simulink model "bmw_vehicle_dynamics"  (R2022b)
settings: Solver=ode45  StartTime=0.0  StopTime=10  RelTol=1e-3  EnableMultiTasking=on
PreLoadFcn:
  | % Execute script to load parameters
  | bmwParams;
values from neighbouring files (symbols this model uses):
  CD = 0.3    [ballParams.m]    (also in bmwParams.m = 0.4; bungeeParams.m = 0.6)
  Fdrive = 1000    [bmwParams.m]
  h = 4.15    [bmwParams.m]
  m = 0.145    [ballParams.m]    (also in bmwParams.m = 104.2; bungeeParams.m = 90)
  rho = 1.2    [ballParams.m]    (also in bmwParams.m = 0.002377; bungeeParams.m)
  w = 5.71    [bmwParams.m]    (also in manifold_press_start.mat = [209.48 209.479999353 209.479996118 209.479979943 209.479899; manifold_pressure.mat = [209.48 209.479999353 209.479996118 209.479979943 209.479899)
settings Model: Creator=jrivitus  LastModifiedBy=bensweet
settings SolverCC: AlgebraicLoopSolver=TrustRegion
settings DataIOCC: LimitDataPoints=on  SaveFormat=Array  ReturnWorkspaceOutputs=off
settings OptimizationCC: ExpressionDepthLimit=2147483647  LifeSpan=inf
settings DebuggingCC: UnderspecifiedInitializationDetection=Classic  MergeDetectMultiDrivingBlocksExec=none  ParameterPrecisionLossMsg=none  FcnCallInpInsideContextMsg=warning  UnconnectedInputMsg=warning  UnconnectedOutputMsg=warning  UnconnectedLineMsg=warning  AllowSymbolicDim=off  StateNameClashWarn=warning  PregeneratedLibrarySubsystemCodeDiagnostic=none  SFUnexpectedBacktrackingDiag=warning  SFNoUnconditionalDefaultTransitionDiag=warning  SFExecutionAtInitializationDiag=none  SFMachineParentedDataDiag=warning  ArithmeticOperatorsInVariantConditions=warning
settings HardwareCC: ProdBitPerPointer=32  ProdBitPerSizeT=32  ProdBitPerPtrDiffT=32  ProdLargestAtomicFloat=None  ProdIntDivRoundTo=Undefined  ProdEndianess=Unspecified  ProdWordSize=32  ProdHWDeviceType=32-bit Generic
settings ModelReferenceCC: EnableRefExpFcnMdlSchedulingChecks=on  PropagateSignalLabelsOutOfModel=off
settings SFSimCC: SimUseLocalCustomCode=off
settings RTWCC: RTWUseLocalCustomCode=off  DLArmComputeVersion=19.05
settings CodeAppCC: StateflowObjectComments=on
settings GRTTargetCC: TargetLangStandard=C89/C90 (ANSI)  CombineOutputUpdateFcns=off  GRTInterface=on
settings ConfigComp: CovMetricSettings=dw  CovSaveCumulativeToWorkspaceVar=on  CovSaveSingleToWorkspaceVar=on  CovExternalEMLEnable=off  CovSFcnEnable=off

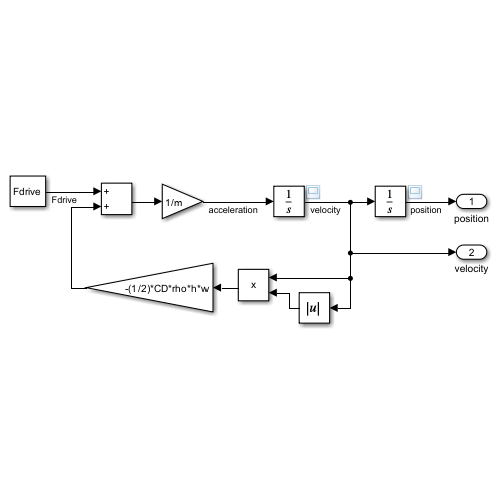
[thumbnail: Simulink's stored preview of the top-level diagram]
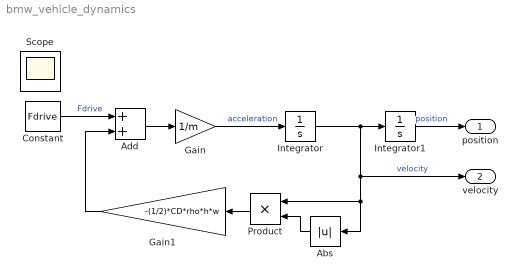
== system bmw_vehicle_dynamics ==
  Abs : Abs  SaturateOnIntegerOverflow=off
  Add : Sum
  Constant : Constant  Value=Fdrive
  Gain : Gain  Gain=1/m
  Gain1 : Gain  Gain=-(1/2)*CD*rho*h*w
  Integrator : Integrator
  Integrator1 : Integrator
  Product : Product  RndMeth=Zero
  position : Outport  VectorParamsAs1DForOutWhenUnconnected=off
  velocity : Outport  Port=2  VectorParamsAs1DForOutWhenUnconnected=off
  Scope : Scope
  wires:
  Constant/1 -> Add/1  "Fdrive"
  Integrator/1 -> Product/1, Abs/1, velocity/1, Integrator1/1  "velocity"
  Integrator1/1 -> position/1  "position"
  Add/1 -> Gain/1
  Gain/1 -> Integrator/1  "acceleration"
  Abs/1 -> Product/2
  Product/1 -> Gain1/1
  Gain1/1 -> Add/2
